simulink model "TST_CoME_DemCoord"  (R2016b)
settings: Solver=FixedStepDiscrete  StartTime=0.0  StopTime=simTime  FixedStep=sampleTime  RelTol=1e-3
values from neighbouring files (symbols this model uses):
  testCase = 1    [initTST_CoME_DemCoord_001.m]    (also in initTST_CoME_DemCoord_002.m = 2; initTST_CoME_DemCoord_003.m = 3; initTST_CoME_DemCoord_004.m = 4)
libraries: simulink x29, UnitTest_Lib x24
(part 2 of 2)

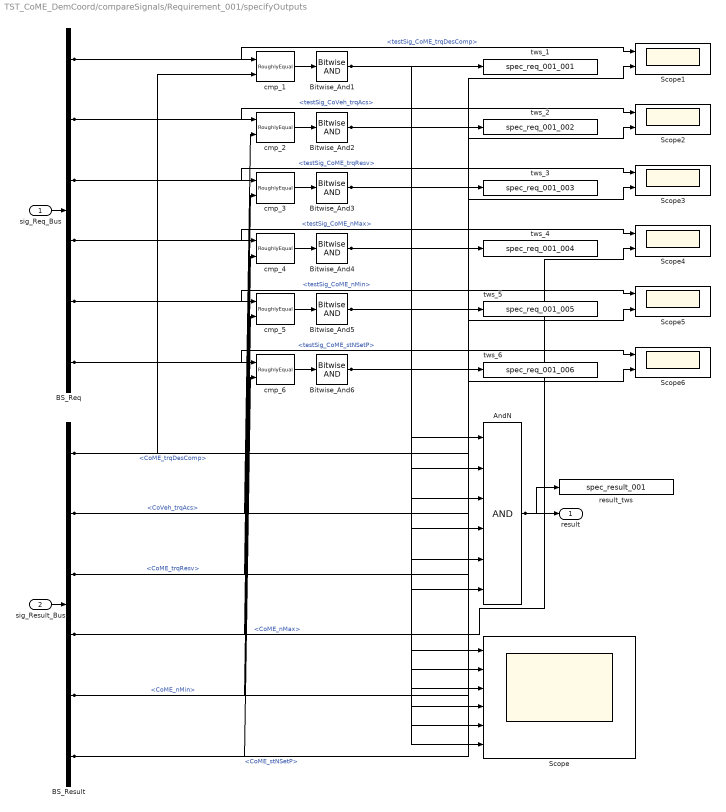
== system TST_CoME_DemCoord/compareSignals/Requirement_001/specifyOutputs ==
  sig_Req_Bus : Inport
  sig_Result_Bus : Inport  Port=2
  AndN : Logic  Inputs=6
  BS_Req : BusSelector  OutputSignals=testSig_CoME_trqDesComp,testSig_CoVeh_trqAcs,testSig_CoME_trqResv,testSig_CoME_nMax,testSig_CoME_nMin,testSig_CoME_stNSetP
  BS_Result : BusSelector  OutputSignals=CoME_trqDesComp,CoVeh_trqAcs,CoME_trqResv,CoME_nMax,CoME_nMin,CoME_stNSetP
  Bitwise_And{1..6} (6 alike) : simulink/Logic and Bit Operations/Bitwise Operator  logicop=AND  UseBitMask=off  BitMask=bin2dec('11011001')  BitMaskRealWorld=Stored Integer
  Scope : Scope  NumInputPorts=6
  Scope{1..6} (6 alike) : Scope  NumInputPorts=2
  cmp_{1..6} (6 alike) : UnitTest_Lib/RoughlyEqual  slope=0.1
  result_tws : ToWorkspace  VariableName=spec_result_001
  tws_1 : ToWorkspace  VariableName=spec_req_001_001
  tws_2 : ToWorkspace  VariableName=spec_req_001_002
  tws_3 : ToWorkspace  VariableName=spec_req_001_003
  tws_4 : ToWorkspace  VariableName=spec_req_001_004
  tws_5 : ToWorkspace  VariableName=spec_req_001_005
  tws_6 : ToWorkspace  VariableName=spec_req_001_006
  result : Outport
  wires:
  sig_Req_Bus/1 -> BS_Req/1
  sig_Result_Bus/1 -> BS_Result/1
  AndN/1 -> result/1, result_tws/1
  BS_Req/1 -> cmp_1/1, Scope1/1  "<testSig_CoME_trqDesComp>"
  BS_Result/1 -> cmp_1/2, Scope1/2  "<CoME_trqDesComp>"
  cmp_1/1 -> Bitwise_And1/1
  Bitwise_And1/1 -> tws_1/1, AndN/1, Scope/1
  BS_Req/2 -> cmp_2/1, Scope2/1  "<testSig_CoVeh_trqAcs>"
  BS_Result/2 -> cmp_2/2, Scope2/2  "<CoVeh_trqAcs>"
  cmp_2/1 -> Bitwise_And2/1
  Bitwise_And2/1 -> tws_2/1, AndN/2, Scope/2
  BS_Req/3 -> cmp_3/1, Scope3/1  "<testSig_CoME_trqResv>"
  BS_Result/3 -> cmp_3/2, Scope3/2  "<CoME_trqResv>"
  cmp_3/1 -> Bitwise_And3/1
  Bitwise_And3/1 -> tws_3/1, AndN/3, Scope/3
  BS_Req/4 -> cmp_4/1, Scope4/1  "<testSig_CoME_nMax>"
  BS_Result/4 -> cmp_4/2, Scope4/2  "<CoME_nMax>"
  cmp_4/1 -> Bitwise_And4/1
  Bitwise_And4/1 -> tws_4/1, AndN/4, Scope/4
  BS_Req/5 -> cmp_5/1, Scope5/1  "<testSig_CoME_nMin>"
  BS_Result/5 -> cmp_5/2, Scope5/2  "<CoME_nMin>"
  cmp_5/1 -> Bitwise_And5/1
  Bitwise_And5/1 -> tws_5/1, AndN/5, Scope/5
  BS_Req/6 -> cmp_6/1, Scope6/1  "<testSig_CoME_stNSetP>"
  BS_Result/6 -> cmp_6/2, Scope6/2  "<CoME_stNSetP>"
  cmp_6/1 -> Bitwise_And6/1
  Bitwise_And6/1 -> tws_6/1, AndN/6, Scope/6

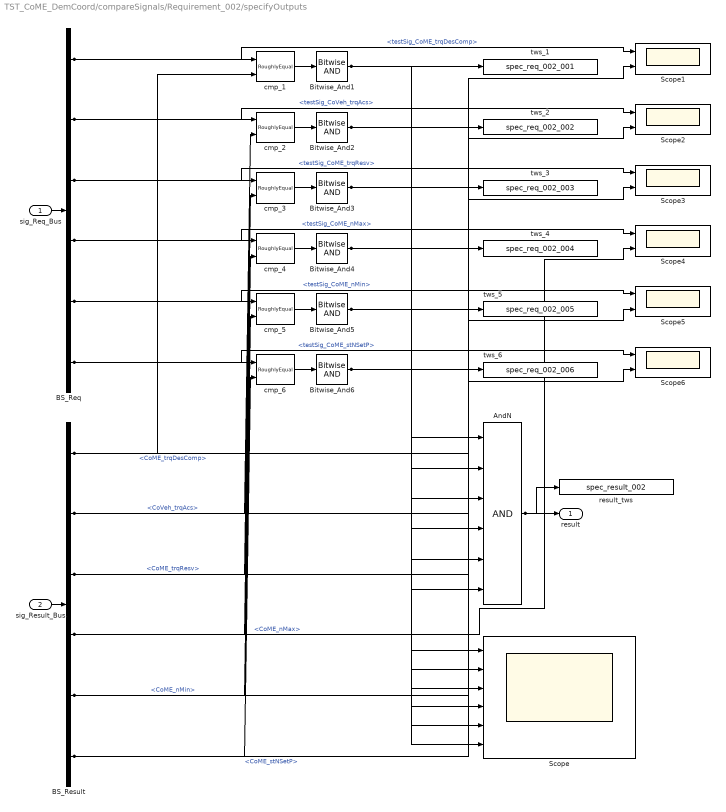
== system TST_CoME_DemCoord/compareSignals/Requirement_002/specifyOutputs ==
  sig_Req_Bus : Inport
  sig_Result_Bus : Inport  Port=2
  AndN : Logic  Inputs=6
  BS_Req : BusSelector  OutputSignals=testSig_CoME_trqDesComp,testSig_CoVeh_trqAcs,testSig_CoME_trqResv,testSig_CoME_nMax,testSig_CoME_nMin,testSig_CoME_stNSetP
  BS_Result : BusSelector  OutputSignals=CoME_trqDesComp,CoVeh_trqAcs,CoME_trqResv,CoME_nMax,CoME_nMin,CoME_stNSetP
  Bitwise_And{1..6} (6 alike) : simulink/Logic and Bit Operations/Bitwise Operator  logicop=AND  UseBitMask=off  BitMask=bin2dec('11011001')  BitMaskRealWorld=Stored Integer
  Scope : Scope  NumInputPorts=6
  Scope{1..6} (6 alike) : Scope  NumInputPorts=2
  cmp_{1..6} (6 alike) : UnitTest_Lib/RoughlyEqual  slope=0.1
  result_tws : ToWorkspace  VariableName=spec_result_002
  tws_1 : ToWorkspace  VariableName=spec_req_002_001
  tws_2 : ToWorkspace  VariableName=spec_req_002_002
  tws_3 : ToWorkspace  VariableName=spec_req_002_003
  tws_4 : ToWorkspace  VariableName=spec_req_002_004
  tws_5 : ToWorkspace  VariableName=spec_req_002_005
  tws_6 : ToWorkspace  VariableName=spec_req_002_006
  result : Outport
  wires:
  sig_Req_Bus/1 -> BS_Req/1
  sig_Result_Bus/1 -> BS_Result/1
  AndN/1 -> result/1, result_tws/1
  BS_Req/1 -> cmp_1/1, Scope1/1  "<testSig_CoME_trqDesComp>"
  BS_Result/1 -> cmp_1/2, Scope1/2  "<CoME_trqDesComp>"
  cmp_1/1 -> Bitwise_And1/1
  Bitwise_And1/1 -> tws_1/1, AndN/1, Scope/1
  BS_Req/2 -> cmp_2/1, Scope2/1  "<testSig_CoVeh_trqAcs>"
  BS_Result/2 -> cmp_2/2, Scope2/2  "<CoVeh_trqAcs>"
  cmp_2/1 -> Bitwise_And2/1
  Bitwise_And2/1 -> tws_2/1, AndN/2, Scope/2
  BS_Req/3 -> cmp_3/1, Scope3/1  "<testSig_CoME_trqResv>"
  BS_Result/3 -> cmp_3/2, Scope3/2  "<CoME_trqResv>"
  cmp_3/1 -> Bitwise_And3/1
  Bitwise_And3/1 -> tws_3/1, AndN/3, Scope/3
  BS_Req/4 -> cmp_4/1, Scope4/1  "<testSig_CoME_nMax>"
  BS_Result/4 -> cmp_4/2, Scope4/2  "<CoME_nMax>"
  cmp_4/1 -> Bitwise_And4/1
  Bitwise_And4/1 -> tws_4/1, AndN/4, Scope/4
  BS_Req/5 -> cmp_5/1, Scope5/1  "<testSig_CoME_nMin>"
  BS_Result/5 -> cmp_5/2, Scope5/2  "<CoME_nMin>"
  cmp_5/1 -> Bitwise_And5/1
  Bitwise_And5/1 -> tws_5/1, AndN/5, Scope/5
  BS_Req/6 -> cmp_6/1, Scope6/1  "<testSig_CoME_stNSetP>"
  BS_Result/6 -> cmp_6/2, Scope6/2  "<CoME_stNSetP>"
  cmp_6/1 -> Bitwise_And6/1
  Bitwise_And6/1 -> tws_6/1, AndN/6, Scope/6

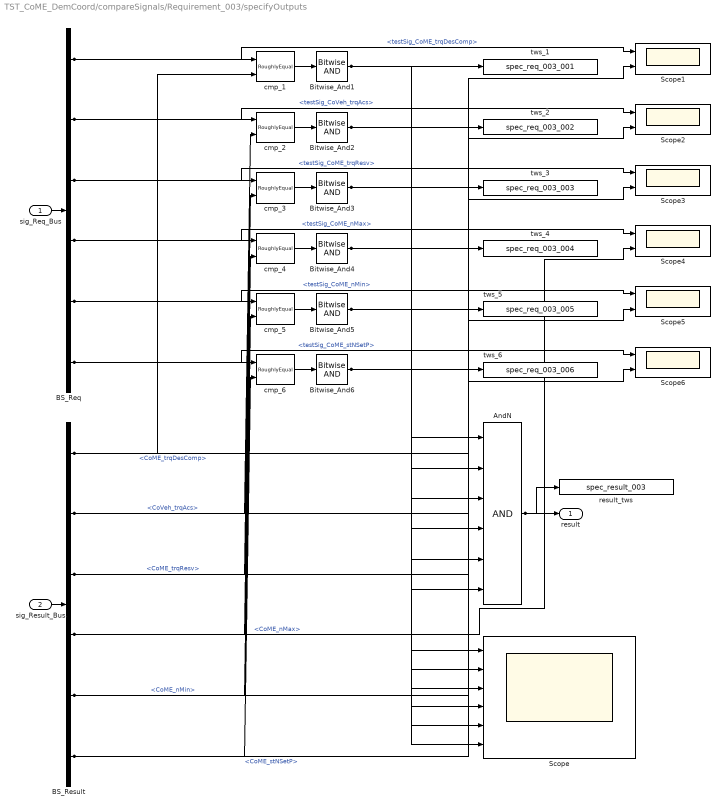
== system TST_CoME_DemCoord/compareSignals/Requirement_003/specifyOutputs ==
  sig_Req_Bus : Inport
  sig_Result_Bus : Inport  Port=2
  AndN : Logic  Inputs=6
  BS_Req : BusSelector  OutputSignals=testSig_CoME_trqDesComp,testSig_CoVeh_trqAcs,testSig_CoME_trqResv,testSig_CoME_nMax,testSig_CoME_nMin,testSig_CoME_stNSetP
  BS_Result : BusSelector  OutputSignals=CoME_trqDesComp,CoVeh_trqAcs,CoME_trqResv,CoME_nMax,CoME_nMin,CoME_stNSetP
  Bitwise_And{1..6} (6 alike) : simulink/Logic and Bit Operations/Bitwise Operator  logicop=AND  UseBitMask=off  BitMask=bin2dec('11011001')  BitMaskRealWorld=Stored Integer
  Scope : Scope  NumInputPorts=6
  Scope{1..6} (6 alike) : Scope  NumInputPorts=2
  cmp_{1..6} (6 alike) : UnitTest_Lib/RoughlyEqual  slope=0.1
  result_tws : ToWorkspace  VariableName=spec_result_003
  tws_1 : ToWorkspace  VariableName=spec_req_003_001
  tws_2 : ToWorkspace  VariableName=spec_req_003_002
  tws_3 : ToWorkspace  VariableName=spec_req_003_003
  tws_4 : ToWorkspace  VariableName=spec_req_003_004
  tws_5 : ToWorkspace  VariableName=spec_req_003_005
  tws_6 : ToWorkspace  VariableName=spec_req_003_006
  result : Outport
  wires:
  sig_Req_Bus/1 -> BS_Req/1
  sig_Result_Bus/1 -> BS_Result/1
  AndN/1 -> result/1, result_tws/1
  BS_Req/1 -> cmp_1/1, Scope1/1  "<testSig_CoME_trqDesComp>"
  BS_Result/1 -> cmp_1/2, Scope1/2  "<CoME_trqDesComp>"
  cmp_1/1 -> Bitwise_And1/1
  Bitwise_And1/1 -> tws_1/1, AndN/1, Scope/1
  BS_Req/2 -> cmp_2/1, Scope2/1  "<testSig_CoVeh_trqAcs>"
  BS_Result/2 -> cmp_2/2, Scope2/2  "<CoVeh_trqAcs>"
  cmp_2/1 -> Bitwise_And2/1
  Bitwise_And2/1 -> tws_2/1, AndN/2, Scope/2
  BS_Req/3 -> cmp_3/1, Scope3/1  "<testSig_CoME_trqResv>"
  BS_Result/3 -> cmp_3/2, Scope3/2  "<CoME_trqResv>"
  cmp_3/1 -> Bitwise_And3/1
  Bitwise_And3/1 -> tws_3/1, AndN/3, Scope/3
  BS_Req/4 -> cmp_4/1, Scope4/1  "<testSig_CoME_nMax>"
  BS_Result/4 -> cmp_4/2, Scope4/2  "<CoME_nMax>"
  cmp_4/1 -> Bitwise_And4/1
  Bitwise_And4/1 -> tws_4/1, AndN/4, Scope/4
  BS_Req/5 -> cmp_5/1, Scope5/1  "<testSig_CoME_nMin>"
  BS_Result/5 -> cmp_5/2, Scope5/2  "<CoME_nMin>"
  cmp_5/1 -> Bitwise_And5/1
  Bitwise_And5/1 -> tws_5/1, AndN/5, Scope/5
  BS_Req/6 -> cmp_6/1, Scope6/1  "<testSig_CoME_stNSetP>"
  BS_Result/6 -> cmp_6/2, Scope6/2  "<CoME_stNSetP>"
  cmp_6/1 -> Bitwise_And6/1
  Bitwise_And6/1 -> tws_6/1, AndN/6, Scope/6

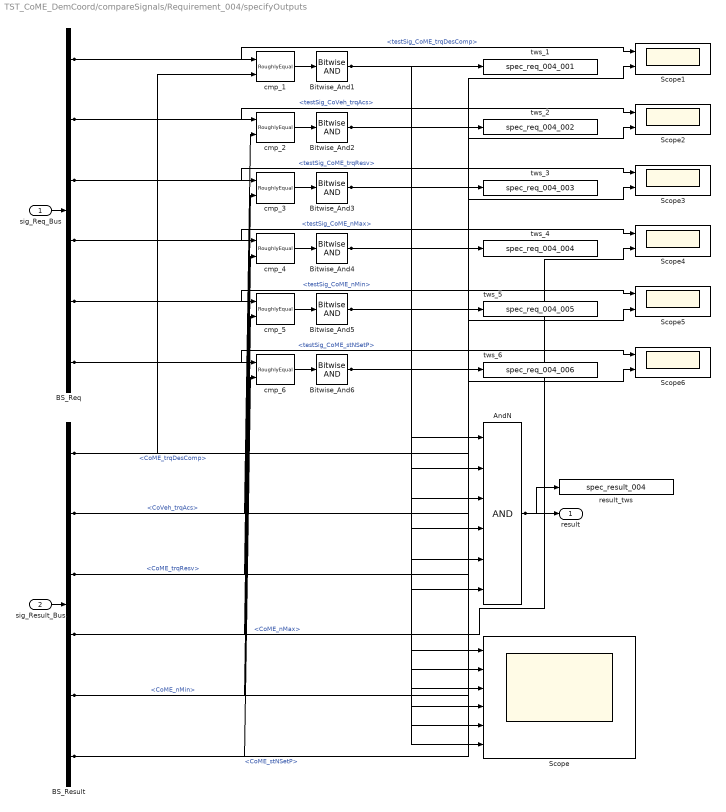
== system TST_CoME_DemCoord/compareSignals/Requirement_004/specifyOutputs ==
  sig_Req_Bus : Inport
  sig_Result_Bus : Inport  Port=2
  AndN : Logic  Inputs=6
  BS_Req : BusSelector  OutputSignals=testSig_CoME_trqDesComp,testSig_CoVeh_trqAcs,testSig_CoME_trqResv,testSig_CoME_nMax,testSig_CoME_nMin,testSig_CoME_stNSetP
  BS_Result : BusSelector  OutputSignals=CoME_trqDesComp,CoVeh_trqAcs,CoME_trqResv,CoME_nMax,CoME_nMin,CoME_stNSetP
  Bitwise_And{1..6} (6 alike) : simulink/Logic and Bit Operations/Bitwise Operator  logicop=AND  UseBitMask=off  BitMask=bin2dec('11011001')  BitMaskRealWorld=Stored Integer
  Scope : Scope  NumInputPorts=6
  Scope{1..6} (6 alike) : Scope  NumInputPorts=2
  cmp_{1..6} (6 alike) : UnitTest_Lib/RoughlyEqual  slope=0.1
  result_tws : ToWorkspace  VariableName=spec_result_004
  tws_1 : ToWorkspace  VariableName=spec_req_004_001
  tws_2 : ToWorkspace  VariableName=spec_req_004_002
  tws_3 : ToWorkspace  VariableName=spec_req_004_003
  tws_4 : ToWorkspace  VariableName=spec_req_004_004
  tws_5 : ToWorkspace  VariableName=spec_req_004_005
  tws_6 : ToWorkspace  VariableName=spec_req_004_006
  result : Outport
  wires:
  sig_Req_Bus/1 -> BS_Req/1
  sig_Result_Bus/1 -> BS_Result/1
  AndN/1 -> result/1, result_tws/1
  BS_Req/1 -> cmp_1/1, Scope1/1  "<testSig_CoME_trqDesComp>"
  BS_Result/1 -> cmp_1/2, Scope1/2  "<CoME_trqDesComp>"
  cmp_1/1 -> Bitwise_And1/1
  Bitwise_And1/1 -> tws_1/1, AndN/1, Scope/1
  BS_Req/2 -> cmp_2/1, Scope2/1  "<testSig_CoVeh_trqAcs>"
  BS_Result/2 -> cmp_2/2, Scope2/2  "<CoVeh_trqAcs>"
  cmp_2/1 -> Bitwise_And2/1
  Bitwise_And2/1 -> tws_2/1, AndN/2, Scope/2
  BS_Req/3 -> cmp_3/1, Scope3/1  "<testSig_CoME_trqResv>"
  BS_Result/3 -> cmp_3/2, Scope3/2  "<CoME_trqResv>"
  cmp_3/1 -> Bitwise_And3/1
  Bitwise_And3/1 -> tws_3/1, AndN/3, Scope/3
  BS_Req/4 -> cmp_4/1, Scope4/1  "<testSig_CoME_nMax>"
  BS_Result/4 -> cmp_4/2, Scope4/2  "<CoME_nMax>"
  cmp_4/1 -> Bitwise_And4/1
  Bitwise_And4/1 -> tws_4/1, AndN/4, Scope/4
  BS_Req/5 -> cmp_5/1, Scope5/1  "<testSig_CoME_nMin>"
  BS_Result/5 -> cmp_5/2, Scope5/2  "<CoME_nMin>"
  cmp_5/1 -> Bitwise_And5/1
  Bitwise_And5/1 -> tws_5/1, AndN/5, Scope/5
  BS_Req/6 -> cmp_6/1, Scope6/1  "<testSig_CoME_stNSetP>"
  BS_Result/6 -> cmp_6/2, Scope6/2  "<CoME_stNSetP>"
  cmp_6/1 -> Bitwise_And6/1
  Bitwise_And6/1 -> tws_6/1, AndN/6, Scope/6
